simulink model "NL_MSD_RefTrajTrac_Opti_FeedBack_Lin_SMC_v01"  (R2024b)
settings: Solver=ode45  StartTime=0.0  StopTime=Tend  FixedStep=Ts  MaxStep=0.001  RelTol=1e-3
values from neighbouring files (symbols this model uses):
  c = zeta * ccr    [Trajectory_Profile_v01.m]
  k = 1e3    (= 1000)    [Trajectory_Profile_v01.m]
  m = 1    [Trajectory_Profile_v01.m]
undefined symbols (not defined in the file or in its folder): aa1, aa2, aa3, eta
libraries: slpidlib x1
settings Model: Creator=ababaei  LastModifiedBy=ababaei
settings SolverCC: AlgebraicLoopSolver=LineSearch
settings DataIOCC: ExternalInput=[spg.setpoint.t, dist.Fz_IH]
settings DebuggingCC: AlgebraicLoopMsg=error  ArtificialAlgebraicLoopMsg=none  UnconnectedInputMsg=warning  UnconnectedOutputMsg=warning  UnconnectedLineMsg=warning  ArithmeticOperatorsInVariantConditions=warning
settings ModelReferenceCC: EnableRefExpFcnMdlSchedulingChecks=on
settings SFSimCC: SimUseLocalCustomCode=off  CustomCodeUndefinedFunction=UseInterfaceOnly
settings RTWCC: RTWUseLocalCustomCode=off  GPUComputeCapability=3.5
settings CodeAppCC: StateflowObjectComments=on

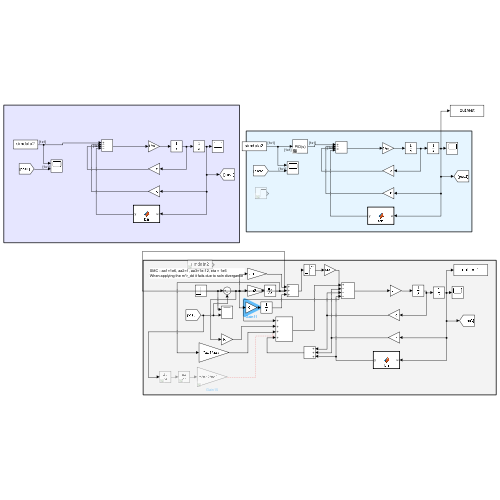
[thumbnail: Simulink's stored preview of the top-level diagram]
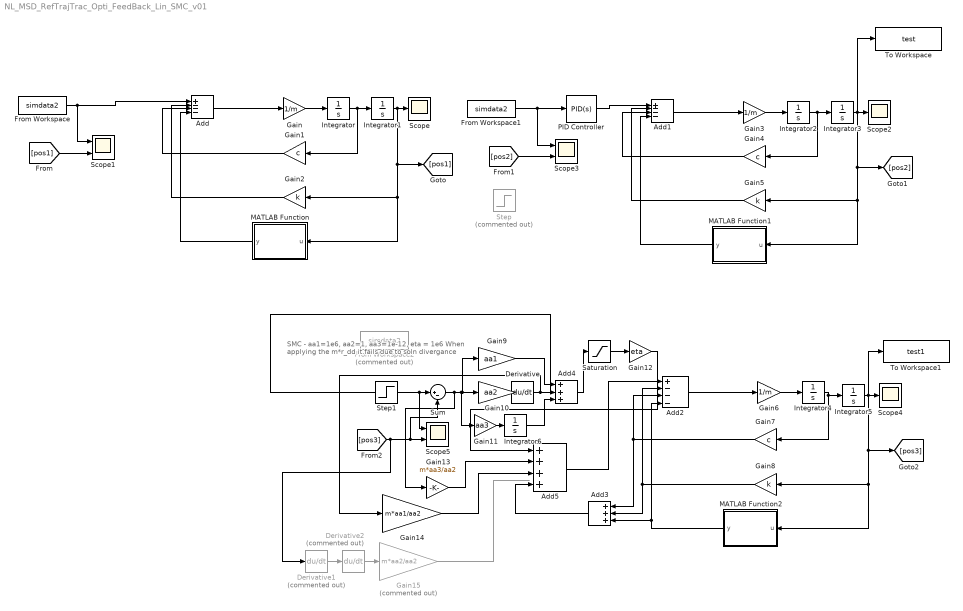
== system NL_MSD_RefTrajTrac_Opti_FeedBack_Lin_SMC_v01 ==
  note: SMC - aa1=1e6, aa2=1, aa3=1e-12, eta = 1e6
      | When applying the m*r_dd it fails due to soln divergance
  Add : Sum  Inputs=+---
  Add1 : Sum  Inputs=+---
  Add2 : Sum  Inputs=+---
  Add3 : Sum  Inputs=+++
  Add4 : Sum  Inputs=+++
  Add5 : Sum  Inputs=++++
  Derivative : Derivative
  Derivative1 : Derivative  Commented=on
  Derivative2 : Derivative  Commented=on
  From Workspace : FromWorkspace  VariableName=simdata2
  From Workspace1 : FromWorkspace  VariableName=simdata2
  From Workspace2 : FromWorkspace  Commented=on  VariableName=simdata2
  Gain : Gain  Gain=1/m
  Gain1 : Gain  Gain=c
  Gain10 : Gain  Gain=aa2
  Gain11 : Gain  Gain=aa3
  Gain12 : Gain  Gain=eta
  Gain13 : Gain  Gain=m*aa3/aa2
  Gain14 : Gain  Gain=m*aa1/aa2
  Gain15 : Gain  Commented=on  Gain=m*aa2/aa2
  Gain2 : Gain  Gain=k
  Gain3 : Gain  Gain=1/m
  Gain4 : Gain  Gain=c
  Gain5 : Gain  Gain=k
  Gain6 : Gain  Gain=1/m
  Gain7 : Gain  Gain=c
  Gain8 : Gain  Gain=k
  Gain9 : Gain  Gain=aa1
  Integrator{,1..6} (7 alike) : Integrator
  MATLAB Function : MATLAB Function  TreatAsAtomicUnit=on
  MATLAB Function1 : MATLAB Function  TreatAsAtomicUnit=on
  MATLAB Function2 : MATLAB Function  TreatAsAtomicUnit=on
  PID Controller : slpidlib/PID Controller  Controller=PID  Form=Parallel  TimeDomain=Continuous-time  UseExternalTs=off  SampleTime=-1  IntegratorMethod=Forward Euler  FilterMethod=Forward Euler  ControllerParametersSource=internal  P=100  I=0  UseKiTs=off  D=0  UseExternalDerivativeSource=off  N=100  UseFilter=on  TunerSelectOption=Transfer Function Based (PID Tuner App)  InitialConditionSource=internal  InitialConditionForIntegrator=0  InitialConditionForFilter=0  DifferentiatorICPrevScaledInput=0  ExternalReset=none  TrackingMode=off  Kt=1  LimitOutput=off  SatLimitsSource=internal  UpperSaturationLimit=inf  LowerSaturationLimit=-inf  LinearizeAsGain=on  AntiWindupMode=none  Kb=1  LimitIntegrator=off  UpperIntegratorSaturationLimit=inf  LowerIntegratorSaturationLimit=-inf  POutMin=[]  POutMax=[]  IOutMin=[]  IOutMax=[]  DOutMin=[]  DOutMax=[]  NOutMin=[]  NOutMax=[]  SumOutMin=[]  SumOutMax=[]  SaturationOutMin=[]  SaturationOutMax=[]  PParamMin=[]  PParamMax=[]  IParamMin=[]  IParamMax=[]  DParamMin=[]  DParamMax=[]  NParamMin=[]  NParamMax=[]  KbParamMin=[]  KbParamMax=[]  KtParamMin=[]  KtParamMax=[]  KbOutMin=[]  KbOutMax=[]  KtOutMin=[]  KtOutMax=[]  IntegratorOutMin=[]  IntegratorOutMax=[]  FilterOutMin=[]  FilterOutMax=[]  SumI1OutMin=[]  SumI1OutMax=[]  SumI2OutMin=[]  SumI2OutMax=[]  SumI3OutMin=[]  SumI3OutMax=[]  SumI4OutMin=[]  SumI4OutMax=[]  SumDOutMin=[]  SumDOutMax=[]  DifferentiatorOutMin=[]  DifferentiatorOutMax=[]  FilterDiffOutCoefMin=[]  FilterDiffOutCoefMax=[]  ReciprocalOutMin=[]  ReciprocalOutMax=[]  SumDenOutMin=[]  SumDenOutMax=[]  SumNumOutMin=[]  SumNumOutMax=[]  DivideOutMin=[]  DivideOutMax=[]  UdiffTsProdOutMin=[]  UdiffTsProdOutMax=[]  NTsProdOutMin=[]  NTsProdOutMax=[]  UintegralTsProdOutMin=[]  UintegralTsProdOutMax=[]  UngainTsProdOutMin=[]  UngainTsProdOutMax=[]  ClampingZeroOutDataTypeStr=Inherit: Inherit via back propagation  ClampingZeroOutMin=[]  ClampingZeroOutMax=[]  FilterDenConstantOutDataTypeStr=Inherit: Inherit via back propagation  FilterDenConstantOutMin=[]  FilterDenConstantOutMax=[]  PCopyOutDataTypeStr=Inherit: Inherit via back propagation  PCopyOutMin=[]  PCopyOutMax=[]  NCopyOutDataTypeStr=Inherit: Inherit via back propagation  NCopyOutMin=[]  NCopyOutMax=[]  IntegratorContinuousStateAttributes=''  IntegratorStateMustResolveToSignalObject=off  IntegratorRTWStateStorageClass=Auto  FilterContinuousStateAttributes=''  FilterStateMustResolveToSignalObject=off  FilterRTWStateStorageClass=Auto  ParallelPVariant=InternalParameters  IdealPVariant=Disabled  IVariant=InternalParameters  DVariant=InternalParameters  IntegratorVariant=Continuous  SatVariant=Disabled  AWVariant=Passthrough  PCopyVariant=Disabled  TRVariant=Disabled  FdbkBlocksVariant=Forward  IdealPFdbkVariant=Disabled  SatFdbkVariant=Disabled  DerivativeFilterVariant=ContFilter  NVariant=InternalParameters  NCopyVariant=Disabled  FilterICVariant=InternalICsFilter  IntegratorICVariant=InternalICs  ExternalResetVariant=Disabled  TRSumVariant=Passthrough  SumFdbkVariant=Disabled  SumVariant=Sum_PID  TsampFilterVariant=InternalTs  TsampNgainVariant=Passthrough  TsampIntegralVariant=Disabled_SignalSpec  ExternalSaturationOutDataTypeStr=Inherit: Same as second input  DerivativeSourceVariant=ErrorSignal  PreIntVariant=InternalPreInt
  Saturation : Saturate
  Scope : Scope
  Scope1 : Scope  NumInputPorts=2
  Scope2 : Scope
  Scope3 : Scope  NumInputPorts=2
  Scope4 : Scope
  Scope5 : Scope  NumInputPorts=2
  Step : Step  Commented=on  Time=0.1  SampleTime=0
  Step1 : Step  Time=0.2  SampleTime=0
  Sum : Sum  Inputs=|+-
  To Workspace : ToWorkspace  VariableName=test  SaveFormat=Timeseries  SampleTime=-1
  To Workspace1 : ToWorkspace  VariableName=test1  SaveFormat=Timeseries  SampleTime=-1
  wires:
  Integrator1/1 -> [pos1], MATLAB Function/1(u), Gain2/1, Scope/1
  Integrator/1 -> Gain1/1, Integrator1/1
  Gain/1 -> Integrator/1
  MATLAB Function/1(y) -> Add/4
  Add/1 -> Gain/1
  Gain1/1 -> Add/3
  Gain2/1 -> Add/2
  From Workspace/1 -> Scope1/1, Add/1
  [pos1] -> Scope1/2
  Integrator3/1 -> To Workspace/1, [pos2], MATLAB Function1/1(u), Gain5/1, Scope2/1
  Gain3/1 -> Integrator2/1
  Add1/1 -> Gain3/1
  From Workspace1/1 -> PID Controller/1, Scope3/1
  Gain5/1 -> Add1/2
  Gain4/1 -> Add1/3
  Integrator2/1 -> Gain4/1, Integrator3/1
  MATLAB Function1/1(y) -> Add1/4
  [pos2] -> Scope3/2
  PID Controller/1 -> Add1/1
  Step1/1 -> Scope5/1, Sum/1
  Gain6/1 -> Integrator4/1
  Integrator5/1 -> To Workspace1/1, [pos3], MATLAB Function2/1(u), Gain8/1, Scope4/1
  Gain8/1 -> Add3/2, Add2/2
  Integrator4/1 -> Gain7/1, Integrator5/1
  MATLAB Function2/1(y) -> Add3/3, Add2/4
  Add2/1 -> Gain6/1
  Add5/1 -> Add2/1
  [pos3] -> Derivative1/1, Sum/2, Scope5/2
  Gain7/1 -> Add3/1, Add2/3
  Sum/1 -> Gain13/1, Gain11/1, Gain9/1, Gain10/1
  Gain11/1 -> Integrator6/1
  Gain10/1 -> Derivative/1
  Derivative/1 -> Gain14/1, Add4/2
  Gain9/1 -> Add4/1
  Integrator6/1 -> Add4/3
  Add4/1 -> Saturation/1
  Saturation/1 -> Gain12/1
  Gain13/1 -> Add5/2
  Gain12/1 -> Add5/1
  Gain14/1 -> Add5/3
  Add3/1 -> Add5/4
  Derivative1/1 -> Derivative2/1
  Derivative2/1 -> Gain15/1
  Gain15/1 -> ?

== matlab function NL_MSD_RefTrajTrac_Opti_FeedBack_Lin_SMC_v01/MATLAB Function ==
  data: u input; y output
function y = fcn(u)
kNL = 0;
y = kNL*u;

== matlab function NL_MSD_RefTrajTrac_Opti_FeedBack_Lin_SMC_v01/MATLAB Function2 ==
  data: u input; y output
function y = fcn(u)
kNL = 100;
y = kNL*u;

== matlab function NL_MSD_RefTrajTrac_Opti_FeedBack_Lin_SMC_v01/MATLAB Function1 ==
  data: u input; y output
function y = fcn(u)
kNL = 100;
y = kNL*u;
